simulink model "BD_CONV"  (Simulink 7.9)
settings: Solver=ode1  SolverMode=SingleTasking  StartTime=0.0  StopTime=max(cyc_mph(:,1))  FixedStep=1  MaxStep=1  RelTol=1e-3  AbsTol=1e-3
undefined symbols (not defined in the file): ess_on, ex_calc, fc_emis, fc_max_trq, fc_trq_scale, vc_idle_bool, vc_idle_spd
libraries: lib_transmission x3, lib_wheel x2, lib_help x2, lib_outputs x1, lib_controls x1, lib_interactive x1, lib_accessory x1, lib_drive_cycle x1, lib_exhaust x1, lib_fuel_converter x1, lib_vehicle x1
settings Model: Creator=mokeefe  LastModifiedBy=mokeefe  ExtModeTrigMode=oneshot  ExtModeArmWhenConnect=off
settings Model: ModifiedComment=|
  | mokeefe -- Thu Apr 18 07:47:12 2002 -- Version 1.98
  | saving the model:
  | o "without the model browser open"
  | o with only top-level screen visible
  | o and with "fit to view" enabled
settings Model: ModifiedHistory=|
  | mokeefe -- Thu Apr 18 07:47:12 2002 -- Version 1.98
  | saving the model:
  | o "without the model browser open"
  | o with only top-level screen visible
  | o and with "fit to view" enabled
  | 
  | mokeefe -- Thu Apr 18 07:46:46 2002 -- Version 1.97
  | saving the model:
  | o "without the model browser open"
  | o with only top-level screen visible
  | o and with "fit to view" enabled
  | 
  | mokeefe -- Thu Apr 18 07:37:24 2002 -- Version 1.96
  | saving the model
  | "without the model browser open"
  | with only top-level screen visible
  | and with "fit to view" enabled
  | 
  | abrooker -- Fri Apr 12 08:11:12 2002 -- Version 1.95
  | 
  | 
  | abrooker -- Fri Apr 12 08:02:30 2002 -- Version 1.94
  | 
  | 
  | abrooker -- Fri Apr 12 08:02:26 2002 -- Version 1.93
  | 
  | 
  | abrooker -- Fri Apr 12 07:59:19 2002 -- Version 1.92
  | 
  | 
  | abrooker -- Fri Apr 12 07:49:13 2002 -- Version 1.91
  | 
  | 
  | mokeefe -- Fri Mar 29 15:46:36 2002 -- Version 1.90
  | 
  | 
  | mokeefe -- Wed Mar 06 11:56:56 2002 -- Version 1.89
  | 
  | 
  | mokeefe -- Wed Mar 06 11:56:30 2002 -- Version 1.88
  | changed the acc_on flag in mechanical accessory loads
  | 
  | mokeefe -- Tue Mar 05 14:28:10 2002 -- Version 1.87
  | 
  | 
  | mokeefe -- Mon Mar 04 14:59:21 2002 -- Version 1.86
  | changed engine_on to key_on in Mechanical Accessory Loads <acc>
  | 
  | mokeefe -- Mon Mar 04 07:29:42 2002 -- Version 1.85
  | 
  | 
  | mokeefe -- Mon Mar 04 07:29:35 2002 -- Version 1.84
  | 
  | 
  | mokeefe -- Fri Mar 01 16:40:39 2002 -- Version 1.83
  | 
  | 
  | mokeefe -- Fri Mar 01 15:08:54 2002 -- Version 1.82
  | 
  | 
  | mokeefe -- Fri Mar 01 12:12:36 2002 -- Version 1.81
  | 
  | 
  | mokeefe -- Fri Mar 01 11:41:50 2002 -- Version 1.80
  | 
  | 
  | mokeefe -- Fri Mar 01 11:21:25 2002 -- Version 1.79
  | 
  | 
  | mokeefe -- Fri Mar 01 10:51:16 2002 -- Version 1.78
  | 
  | 
  | mokeefe -- Fri Mar 01 10:28:03 2002 -- Version 1.77
  | 
  | 
  | mokeefe -- Fri Mar 01 10:27:49 2002 -- Version 1.76
  | 
  | 
  | mokeefe -- Fri Mar 01 10:27:36 2002 -- Version 1.75
  | 
  | 
  | mokeefe -- Thu Feb 28 08:54:13 2002 -- Version 1.74
  | 
  | 
  | mokeefe -- Thu Feb 28 08:41:46 2002 -- Version 1.73
  | 
  | 
  | mokeefe -- Thu Feb 28 08:40:29 2002 -- Version 1.72
  | 
  | 
  | mokeefe -- Thu Feb 28 08:37:03 2002 -- Version 1.71
  | 
  | 
  | mokeefe -- Thu Feb 28 08:29:13 2002 -- Version 1.70
  | changing the mechanical auxiliary loads block to be more simplistic
  | 
  | mokeefe -- Wed Feb 27 14:39:18 2002 -- Version 1.69
  | 
  | 
  | mokeefe -- Wed Feb 27 14:38:57 2002 -- Version 1.68
  | 
  | 
  | mokeefe -- Wed Feb 27 14:16:01 2002 -- Version 1.67
  | changing to Mechanical Accessory Loads v2 <acc> from lib_accessory
  | 
  | mokeefe -- Wed Feb 27 14:14:56 2002 -- Version 1.66
  | 
  | 
  | mokeefe -- Tue Feb 26 10:43:51 2002 -- Version 1.65
  | changing the way that the auxiliary loads are calculated and logged to workspace. Electrical loads run on a conventional powertrain are assumed to have a mechanical to electrical efficiency penalty but are translated and added as mechanical loads
  | 
  | mokeefe -- Tue Feb 26 10:36:09 2002 -- Version 1.64
  | 
  | 
  | mokeefe -- Tue Feb 26 09:51:22 2002 -- Version 1.63
  | changed the condition for whether electrical loads are accounted in auxiliary loads block (Mechanical Accessory Loads <acc>) to be not(ess_on)
  | 
  | mokeefe -- Mon Feb 25 15:04:18 2002 -- Version 1.62
  | 
  | 
  | mokeefe -- Mon Feb 25 14:59:54 2002 -- Version 1.61
  | 
  | 
  | mokeefe -- Mon Feb 25 14:24:21 2002 -- Version 1.60
  | 
  | 
  | mokeefe -- Fri Feb 15 11:53:40 2002 -- Version 1.59
  | added and tested  Mechanical Accessory Loads <acc> block
  | 
  | mokeefe -- Thu Feb 14 17:56:13 2002 -- Version 1.58
  | 
  | 
  | mokeefe -- Thu Feb 14 17:21:52 2002 -- Version 1.57
  | 
  | 
  | mokeefe -- Thu Feb 14 17:05:06 2002 -- Version 1.56
  | updated with Mechanical Accessory Loads <acc> block
  | 
  | mokeefe -- Thu Feb 14 16:31:11 2002 -- Version 1.55
  | 
  | 
  | mokeefe -- Thu Feb 14 16:04:04 2002 -- Version 1.54
  | added Mechanical Auxiliary Loads (acc) block
  | 
  | mokeefe -- Thu Feb 14 10:48:35 2002 -- Version 1.53
  | 
  | 
  | mokeefe -- Thu Feb 14 10:41:17 2002 -- Version 1.52
  | 
  | 
  | mokeefe -- Thu Feb 14 10:24:42 2002 -- Version 1.51
  | 
  | 
  | mokeefe -- Thu Feb 14 09:59:11 2002 -- Version 1.50
  | testing
  | 
  | 
  | ssprik -- Fri Feb 09 15:14:35 2001 -- Version 1.49
  | changed foregrounds to black colors
settings DataIOCC: LimitDataPoints=off  SaveOutput=off  SaveTime=off
settings OptimizationCC: BooleanDataType=off
settings DebuggingCC: SaveWithParameterizedLinksMsg=none  SignalResolutionControl=TryResolveAllWithWarning  SolverPrmCheckMsg=none  MultiTaskDSMMsg=warning  MultiTaskCondExecSysMsg=none  UnconnectedLineMsg=none  StrictBusMsg=None
settings HardwareCC: TargetUnknown=on
settings RTWCC: TemplateMakefile=grt_vc.tmf  IncludeERTFirstTime=on
settings GRTTargetCC: CombineOutputUpdateFcns=off  GRTInterface=on

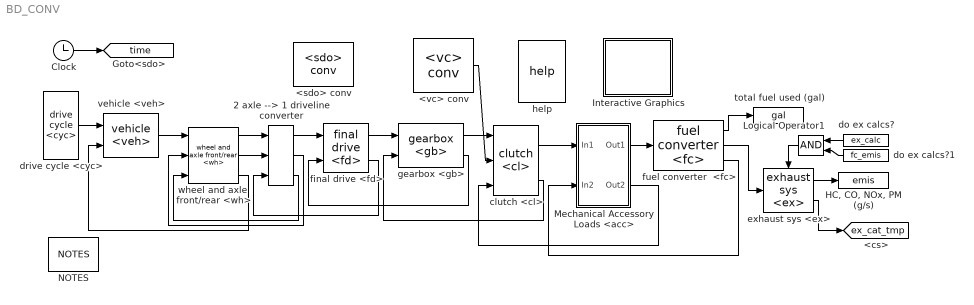
== system BD_CONV ==
  2 axle --> 1 driveline converter : lib_wheel/2 axle --> 1 driveline converter
  <sdo> conv : lib_outputs/<sdo> conv  SystemSampleTime=-1
  <vc> conv : lib_controls/<vc> conv  SystemSampleTime=-1
      link override config traction control: BlockChoice=traction control 2 axle
  Clock : Clock
  "HC, CO, NOx, PM (g/s)" : ToWorkspace  VariableName=emis
  Interactive Graphics : Subsystem  BlockChoice=off
      settings: AttributesFormatString=%<BlockChoice>  TemplateBlock=lib_interactive/Interactive Graphics  MemberBlocks=off,on
  Logical Operator1 : Logic
  Mechanical Accessory Loads <acc> : Subsystem
      mask Display: image(imread('bdi_acc_pic.bmp'))
  NOTES : lib_help/NOTES  SystemSampleTime=-1
  clutch <cl> : lib_transmission/clutch <cl>  slip_spd=vc_launch_spd  maxtrq=max(fc_max_trq)*fc_trq_scale
  do ex calcs? : Constant  Value=ex_calc
  do ex calcs?1 : Constant  Value=fc_emis
  drive cycle <cyc> : lib_drive_cycle/drive cycle <cyc>  SystemSampleTime=-1
  exhaust sys <ex> : lib_exhaust/exhaust sys <ex>  SystemSampleTime=-1
  final drive <fd> : lib_transmission/final drive <fd>  SystemSampleTime=-1
  fuel converter  <fc> : lib_fuel_converter/fuel converter  <fc>  SystemSampleTime=-1
      link override fuel use and EO emis Configurable Subsystem: BlockChoice=fuel use and EO emis
  gearbox <gb> : lib_transmission/gearbox <gb>  SystemSampleTime=-1
  help : lib_help/help  SystemSampleTime=-1
  total fuel used (gal) : ToWorkspace  VariableName=gal
  vehicle <veh> : lib_vehicle/vehicle <veh>  SystemSampleTime=-1
      link override record achieved force outputs/rolling resistance force: BlockChoice=force req'd to overcome rolling resistance (N)
      link override rolling resistance force: BlockChoice=force req'd to overcome rolling resistance (N)
      link override vehicle speed: BlockChoice=vehicle speed (m/s)
  wheel and axle  front/rear <wh> : lib_wheel/wheel and axle  front//rear <wh>  SystemSampleTime=-1
  tag scope: ex_cat_tmp=global, time=global
  wires:
  Clock/1 -> [time]
  final drive <fd>/1 -> gearbox <gb>/1
  gearbox <gb>/2 -> final drive <fd>/2
  drive cycle <cyc>/1 -> vehicle <veh>/1
  vehicle <veh>/1 -> wheel and axle  front/rear <wh>/1
  gearbox <gb>/1 -> clutch <cl>/1
  clutch <cl>/2 -> gearbox <gb>/2
  <vc> conv/1 -> clutch <cl>/2
  fuel converter  <fc>/2 -> exhaust sys <ex>/1
  fuel converter  <fc>/1 -> total fuel used (gal)/1
  exhaust sys <ex>/1 -> "HC, CO, NOx, PM (g/s)"/1
  Logical Operator1/1 -> exhaust sys <ex>/Enable
  do ex calcs?/1 -> Logical Operator1/1
  do ex calcs?1/1 -> Logical Operator1/2
  exhaust sys <ex>/2 -> [ex_cat_tmp]
  clutch <cl>/1 -> Mechanical Accessory Loads <acc>/1(In1)
  Mechanical Accessory Loads <acc>/1(Out1) -> fuel converter  <fc>/1
  fuel converter  <fc>/3 -> Mechanical Accessory Loads <acc>/2(In2)
  Mechanical Accessory Loads <acc>/2(Out2) -> clutch <cl>/3
  wheel and axle  front/rear <wh>/1 -> 2 axle --> 1 driveline converter/1
  wheel and axle  front/rear <wh>/2 -> 2 axle --> 1 driveline converter/2
  final drive <fd>/2 -> 2 axle --> 1 driveline converter/3
  2 axle --> 1 driveline converter/1 -> final drive <fd>/1
  2 axle --> 1 driveline converter/2 -> wheel and axle  front/rear <wh>/2
  2 axle --> 1 driveline converter/3 -> wheel and axle  front/rear <wh>/3
  wheel and axle  front/rear <wh>/3 -> vehicle <veh>/2

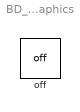
== system BD_CONV/Interactive Graphics ==
  off : lib_interactive/off  Tag=Altia_off  SystemSampleTime=-1

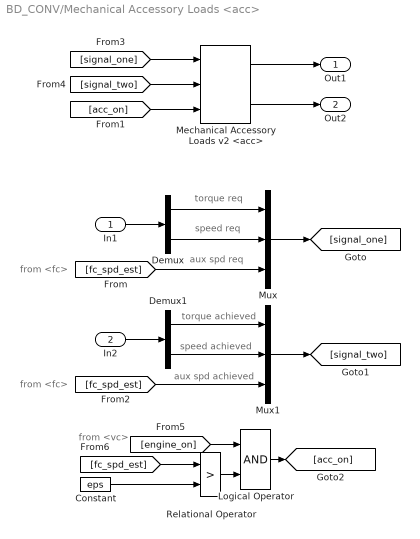
== system BD_CONV/Mechanical Accessory Loads <acc> ==
  note: from <fc>
  note: from <fc>
  note: torque req
  note: speed req
  note: aux spd req
  note: torque achieved
  note: speed achieved
  note: aux spd achieved
  note: from <vc>
  In1 : Inport
  In2 : Inport  Port=2
  Constant : Constant  Value=eps
  Demux : Demux  Outputs=2
  Demux1 : Demux  Outputs=2
  Logical Operator : Logic
  Mechanical Accessory Loads v2 <acc> : lib_accessory/Mechanical Accessory Loads v2 <acc>  load_on=not(ess_on)*1  acc_max_spd=inf  acc_min_spd=(vc_idle_spd*vc_idle_bool)+eps  ic_mech_trq=0  ic_mech_pwr=0
      link override backward model/mechanical accessories (Nm): BlockChoice=Mechanical Accessories: Const Mech Var Elect
  Mux : Mux  Inputs=3
  Mux1 : Mux  Inputs=3
  Relational Operator : RelationalOperator  Operator=>  InputSameDT=on
  Out1 : Outport
  Out2 : Outport  Port=2
  wires:
  [signal_one] -> Mechanical Accessory Loads v2 <acc>/1
  Mechanical Accessory Loads v2 <acc>/1 -> Out1/1
  Mechanical Accessory Loads v2 <acc>/2 -> Out2/1
  [signal_two] -> Mechanical Accessory Loads v2 <acc>/2
  [acc_on] -> Mechanical Accessory Loads v2 <acc>/3
  Mux/1 -> [signal_one]
  In1/1 -> Demux/1
  Demux/1 -> Mux/1
  Demux/2 -> Mux/2
  [fc_spd_est] -> Mux/3
  Mux1/1 -> [signal_two]
  In2/1 -> Demux1/1
  Demux1/1 -> Mux1/1
  Demux1/2 -> Mux1/2
  [fc_spd_est] -> Mux1/3
  [fc_spd_est] -> Relational Operator/1
  Constant/1 -> Relational Operator/2
  [engine_on] -> Logical Operator/1
  Relational Operator/1 -> Logical Operator/2
  Logical Operator/1 -> [acc_on]
